simulink model "Level3"  (R2012b)
settings: Solver=FixedStepDiscrete  StartTime=0.0  StopTime=50  RelTol=1e-3
InitFcn:
  | N=256;
  | Fs = 1000;
  | bw = 5.6;
undefined symbols (not defined in the file): gcbh, rmidispblock, T1, T2
settings Model: RequirementInfo={'other' '..\..\..\requirements\ebd_srs.doc' '@Simulink_requirement_level3' 'true' '3.1.3.4 Level 3 PD' '' } %GIDa_2e90d62d_b465_46ce_8983_35d460f9da2e  Creator=aanantha  LastModifiedBy=klindqvi
settings DataIOCC: SaveFormat=Structure  SignalLoggingSaveFormat=ModelDataLogs  SaveOutput=off  SaveTime=off  SignalLoggingName=logsOut
settings OptimizationCC: InlineParams=on  OptimizeModelRefInitCode=on  LifeSpan=1
settings DebuggingCC: ReadBeforeWriteMsg=DisableAll  WriteAfterWriteMsg=DisableAll  WriteAfterReadMsg=DisableAll  SolverPrmCheckMsg=none  InheritedTsInSrcMsg=none  ParameterPrecisionLossMsg=none  FcnCallInpInsideContextMsg=EnableAllAsWarning
settings HardwareCC: ProdLargestAtomicInteger=Long  ProdLargestAtomicFloat=Double  ProdEndianess=LittleEndian  ProdHWDeviceType=ARM Compatible->ARM Cortex
settings RTWCC: SystemTargetFile=ert.tlc  TemplateMakefile=ert_default_tmf  Description=Embedded Coder  GenerateReport=on  RTWVerbose=off  ProcessScript=ert_make_rtw_hook  IncludeHyperlinkInReport=on  LaunchReport=on  PortableWordSizes=on  CodeProfilingSaveOptions=AllData  GenerateTraceInfo=on  GenerateTraceReportSl=on  GenerateTraceReportSf=on  GenerateTraceReportEml=on  GenerateCodeMetricsReport=on
settings CodeAppCC: IgnoreCustomStorageClasses=off
settings ERTTargetCC: CodeReplacementLibrary=GCC ARM Cortex-A8  MultiwordLength=2048  GenerateSampleERTMain=on  ERTCustomFileTemplate=example_file_process.tlc  ConvertIfToSwitch=off  SuppressUnreachableDefaultCases=off

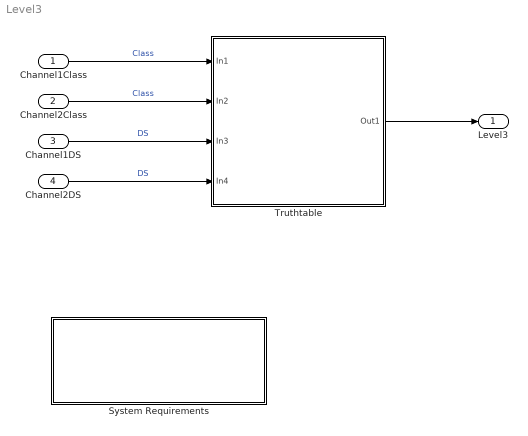
== system Level3 ==
  Channel1Class : Inport  OutDataTypeStr=boolean  PortDimensions=1  SampleTime=[0.08900000000000001,0]
  Channel2Class : Inport  Port=2  OutDataTypeStr=boolean  PortDimensions=1  SampleTime=[0.08900000000000001,0]
  Channel1DS : Inport  Port=3  OutDataTypeStr=double  PortDimensions=1  SampleTime=[0.08900000000000001,0]
  Channel2DS : Inport  Port=4  OutDataTypeStr=double  PortDimensions=1  SampleTime=[0.08900000000000001,0]
  System Requirements : Subsystem  LoadFcn=rmidispblock('load',gcbh)  mask(System Requirements){id=SystemReq, title=System Requirements}
      mask prompts: title "Block Title"
      mask help: Lists the requirements for the current model.
      mask init:
      | id = 'SystemReq';
      | [w,h] = rmidispblock('display',gcbh);
      settings: CopyFcn=rmidispblock('create',gcbh)  DeleteFcn=rmidispblock('delete',gcbh)  ModelCloseFcn=rmidispblock('close',gcbh)  PreSaveFcn=rmidispblock('close',gcbh)  PostSaveFcn=rmidispblock('open',gcbh)  OpenFcn=rmidispblock('open',gcbh)  MoveFcn=rmidispblock('move',gcbh)
      mask Help: helpview(fullfile(docroot,'toolbox','slvnv','slvnv.map'),'systemrequirements')
      mask Display: text(w/2,h-4,rmidispblock('title',gcbh),'horizontalAlignment','center','verticalAlignment','top')
  Truthtable : Subsystem
  Level3 : Outport  OutDataTypeStr=boolean  PortDimensions=1  SampleTime=[0.08900000000000001,0]
  wires:
  Channel1Class/1 -> Truthtable/1(In1)  "Class"
  Channel2Class/1 -> Truthtable/2(In2)  "Class"
  Channel1DS/1 -> Truthtable/3(In3)  "DS"
  Channel2DS/1 -> Truthtable/4(In4)  "DS"
  Truthtable/1(Out1) -> Level3/1

== system Level3/System Requirements ==

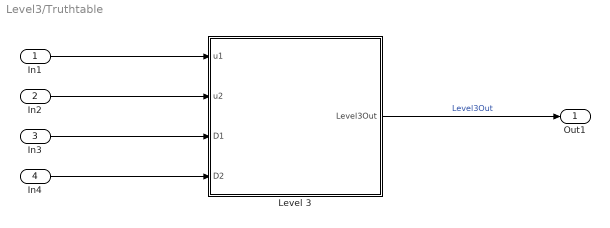
== system Level3/Truthtable ==
  In1 : Inport
  In2 : Inport  Port=2
  In3 : Inport  Port=3
  In4 : Inport  Port=4
  Level 3 : Truth Table  TreatAsAtomicUnit=on
  Out1 : Outport
  wires:
  In4/1 -> Level 3/4(D2)
  In3/1 -> Level 3/3(D1)
  In1/1 -> Level 3/1(u1)
  Level 3/1(Level3Out) -> Out1/1  "Level3Out"
  In2/1 -> Level 3/2(u2)

== matlab function Level3/Truthtable/Level 3 ==
  data: u1 input boolean; Level3Out output; T1 parameter double size=1; T2 parameter double size=1; u2 input boolean; D1 input double size=1; D2 input double size=1
function Level3Out = fcn(u1, T1, T2, u2, D1, D2)

aVarTruthTableCondition_1 = false;
aVarTruthTableCondition_2 = false;


% Channel 1 Beat?

aVarTruthTableCondition_1 = logical(u1 == 1);

% Channel 2 Beat?

aVarTruthTableCondition_2 = logical(u2 == 1);

if (aVarTruthTableCondition_1 && aVarTruthTableCondition_2)
    aFcnTruthTableAction_1();
elseif (~aVarTruthTableCondition_1 && aVarTruthTableCondition_2)
    aFcnTruthTableAction_1();
elseif (~aVarTruthTableCondition_1 && ~aVarTruthTableCondition_2)
    aFcnTruthTableAction_2();
else % Default
    aFcnTruthTableAction_3();
end

function aFcnTruthTableAction_1()

% Output a-Beat

Level3Out = true;

function aFcnTruthTableAction_2()

% Output not-a-beat

Level3Out = false;

function aFcnTruthTableAction_3()

% Calculate D1?D2

if ( (D1-T1)/(1-T1) ) > ( (T2-D2)/(T2) )
Level3Out = true; 
else
Level3Out = false;
end
